simulink library "Lib_MCHP_BLKDEMO_Motor"  (R2015b)
settings: Solver=VariableStepAuto  StartTime=0.0  StopTime=10.0  RelTol=1e-3
values from neighbouring files (symbols this model uses):
  DEADTIME = 1e-6    (= 1e-06)    [UserParams.m]
  PSHIFT = TConv/2    (= 4.680375e-06)    [UserParams.m]
  PWMFREQUENCY = 20e3    (= 20000)    [UserParams.m]
  TSETTLE = 2e-6    (= 2e-06)    [UserParams.m]
  TSmp = 0.343*1e-6    (= 3.43e-07)    [UserParams.m]
undefined symbols (not defined in the file or in its folder): A4, B15, B9, C6, F0, P20, P41, P47, P54, P96, Pin, PWMmax, XData
libraries: MCHP_Blockset x9, simulink x7, Lib_MCHP_BLKDEMO_Motor x6
(part 1 of 2)
settings Model: Creator=M91449  LastModifiedBy=M91449

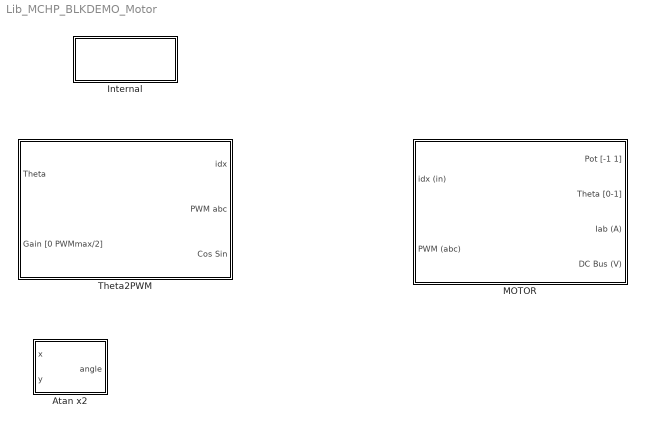
== system Lib_MCHP_BLKDEMO_Motor ==
  Atan x2 : Subsystem
  Internal : Subsystem
  MOTOR : Subsystem  Variant=on  OverrideUsingVariant=SingleShunt_CenterAligned
  Theta2PWM : Subsystem  Variant=on  VariantControl=Variant  OverrideUsingVariant=Optimized

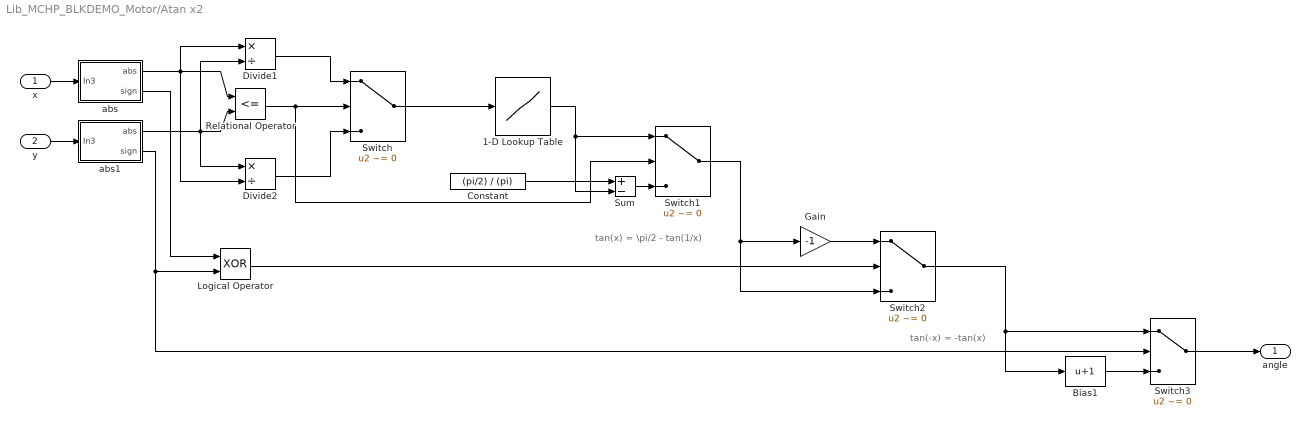
== system Lib_MCHP_BLKDEMO_Motor/Atan x2 ==
  note: tan(x) = \pi/2 - tan(1/x)
  note: tan(-x) = -tan(x)
  x : Inport
  y : Inport  Port=2
  1-D Lookup Table : Lookup_n-D  NumberOfTableDimensions=1  BreakpointsSpecification=Even spacing  BreakpointsForDimension1=[0:2^-8:1]  BreakpointsForDimension1FirstPoint=0  BreakpointsForDimension1Spacing=2^-8  IndexSearchMethod=Evenly spaced points  BeginIndexSearchUsingPreviousIndexResult=on  Table=atan([0:2^-8:1])/(pi)  TableDataTypeStr=fixdt(1,16,15)  InterpMethod=Flat  ExtrapMethod=Clip  RemoveProtectionInput=on  UseLastTableValue=on  OutDataTypeStr=fixdt(1,16,15)  RndMeth=Simplest  InputSameDT=on  LockScale=on
  Bias1 : Bias  Bias=1
  Constant : Constant  Value=(pi/2) / (pi)  OutDataTypeStr=Inherit: Inherit via back propagation
  Divide1 : Product  Inputs=*/  OutDataTypeStr=fixdt(0,16,15)
  Divide2 : Product  Inputs=*/  OutDataTypeStr=fixdt(0,16,15)
  Gain : Gain  Gain=-1  OutDataTypeStr=Inherit: Same as input
  Logical Operator : Logic  Operator=XOR  AllPortsSameDT=off  OutDataTypeStr=boolean
  Relational Operator : RelationalOperator  Operator=<=  OutDataTypeStr=boolean
  Sum : Sum  Inputs=+-
  Switch{,1..3} (4 alike) : Switch  Criteria=u2 ~= 0
  abs : Subsystem
  abs1 : Subsystem
  angle : Outport
  wires:
  Gain/1 -> Switch2/1
  Bias1/1 -> Switch3/3
  Switch3/1 -> angle/1
  Switch2/1 -> Switch3/1, Bias1/1
  Relational Operator/1 -> Switch/2, Switch1/2
  Divide2/1 -> Switch/3
  Divide1/1 -> Switch/1
  Switch/1 -> 1-D Lookup Table/1
  1-D Lookup Table/1 -> Switch1/1, Sum/2
  Constant/1 -> Sum/1
  Sum/1 -> Switch1/3
  abs/1(abs) -> Relational Operator/1, Divide1/1, Divide2/2
  x/1 -> abs/1(In3)
  abs1/1(abs) -> Relational Operator/2, Divide2/1, Divide1/2
  y/1 -> abs1/1(In3)
  abs/2(sign) -> Logical Operator/1
  abs1/2(sign) -> Logical Operator/2, Switch3/2
  Logical Operator/1 -> Switch2/2
  Switch1/1 -> Gain/1, Switch2/3

== system Lib_MCHP_BLKDEMO_Motor/Internal ==
  Trig : Subsystem

== system Lib_MCHP_BLKDEMO_Motor/MOTOR ==
  idx (in) : Inport
  PWM (abc) : Inport  Port=2
  DUAL SHUNT Center Aligned : Subsystem  VariantControl=(default)
  SINGLE SHUNT Center Aligned : Subsystem  VariantControl=SingleShunt_CenterAligned
  SINGLE SHUNT Edge Aligned : Subsystem  VariantControl=SingleShunt_EdgeAligned
  Pot [-1 1] : Outport
  Theta [0-1] : Outport  Port=2
  Iab (A) : Outport  Port=3
  DC Bus (V) : Outport  Port=4

== system Lib_MCHP_BLKDEMO_Motor/Theta2PWM ==
  Theta : Inport
  Gain [0 PWMmax/2] : Inport  Port=2
  Theta2PWM : Subsystem  VariantControl=(default)
  Theta2PWM Optimized : Subsystem  VariantControl=Optimized
  idx : Outport
  PWM abc : Outport  Port=2
  Cos Sin : Outport  Port=3

== system Lib_MCHP_BLKDEMO_Motor/Atan x2/abs ==
  In3 : Inport
  Compare To Zero : simulink/Logic and Bit Operations/Compare To Zero  relop=>=  OutDataTypeStr=boolean
  Gain : Gain  Gain=-1  OutDataTypeStr=Inherit: Same as input
  Switch2 : Switch  Criteria=u2 ~= 0
  abs : Outport
  sign : Outport  Port=2
  wires:
  Compare To Zero/1 -> Switch2/2, sign/1
  In3/1 -> Compare To Zero/1, Switch2/1, Gain/1
  Gain/1 -> Switch2/3
  Switch2/1 -> abs/1

== system Lib_MCHP_BLKDEMO_Motor/Atan x2/abs1 ==
  In3 : Inport
  Compare To Zero : simulink/Logic and Bit Operations/Compare To Zero  relop=>=  OutDataTypeStr=boolean
  Gain : Gain  Gain=-1  OutDataTypeStr=Inherit: Same as input
  Switch2 : Switch  Criteria=u2 ~= 0
  abs : Outport
  sign : Outport  Port=2
  wires:
  Switch2/1 -> abs/1
  Gain/1 -> Switch2/3
  In3/1 -> Gain/1, Switch2/1, Compare To Zero/1
  Compare To Zero/1 -> sign/1, Switch2/2

== system Lib_MCHP_BLKDEMO_Motor/Internal/Trig ==
  note: Compute ADC Trig point for Single Shunt Center Aligned Motor Control drive
  In1 : Inport
  Bias : Bias  Bias=65535-2*PWMmax
  Bias1 : Bias  Bias=65535-2*PWMmax
  Constant1 : Constant  Value=floor(PWMmax + (DEADTIME + TSETTLE - TSmp) * PWMmax * PWMFREQUENCY*2)  OutDataTypeStr=uint16
  Demux8 : Demux  Outputs=2
  Gain : Gain  OutDataTypeStr=Inherit: Same as input
  Mux43 : Mux  Inputs=2
  Sum7 : Sum  OutDataTypeStr=Inherit: Same as accumulator
  Switch : Switch  Criteria=u2 > Threshold  Threshold=2*PWMmax
  Switch1 : Switch  Criteria=u2 > Threshold  Threshold=2*PWMmax
  Out1 : Outport
  wires:
  Bias1/1 -> Switch1/1
  Bias/1 -> Switch/1
  Demux8/1 -> Mux43/1, Bias/1, Switch/2, Switch/3
  Demux8/2 -> Mux43/2, Bias1/1, Switch1/2, Switch1/3
  Gain/1 -> Demux8/1
  In1/1 -> Sum7/2
  Sum7/1 -> Gain/1
  Constant1/1 -> Sum7/1
  Mux43/1 -> Out1/1

== system Lib_MCHP_BLKDEMO_Motor/MOTOR/DUAL SHUNT Center Aligned ==
  idx (in) : Inport
  PWM (abc) : Inport  Port=2
  MOTOR Cmd : Subsystem
  MOTOR - Board Sensor : Subsystem
  Pot [-1 1] : Outport
  Theta [0-1] : Outport  Port=2
  Iab (A) : Outport  Port=3
  DC Bus (V) : Outport  Port=4
  wires:
  MOTOR - Board Sensor/3(Theta) -> Theta [0-1]/1
  MOTOR Cmd/1(idx out) -> MOTOR - Board Sensor/1(idx (in))
  MOTOR - Board Sensor/1(DC Bus (V)) -> DC Bus (V)/1
  MOTOR - Board Sensor/4(Pot) -> Pot [-1 1]/1
  PWM (abc)/1 -> MOTOR Cmd/2(PWM (abc))
  MOTOR - Board Sensor/2(Iab (A)) -> Iab (A)/1
  idx (in)/1 -> MOTOR Cmd/1(idx in)

== system Lib_MCHP_BLKDEMO_Motor/MOTOR/SINGLE SHUNT Center Aligned ==
  idx (in) : Inport
  PWM (abc) : Inport  Port=2
  MOTOR Cmd : Subsystem
  MOTOR - Board Sensor : Subsystem
  Pot [-1 1] : Outport
  Theta [0-1] : Outport  Port=2
  Iab (A) : Outport  Port=3
  DC Bus (V) : Outport  Port=4
  wires:
  idx (in)/1 -> MOTOR Cmd/1(idx in)
  MOTOR - Board Sensor/2(Iab (A)) -> Iab (A)/1
  PWM (abc)/1 -> MOTOR Cmd/2(PWM (abc))
  MOTOR - Board Sensor/4(Pot) -> Pot [-1 1]/1
  MOTOR - Board Sensor/1(DC Bus (V)) -> DC Bus (V)/1
  MOTOR Cmd/1(idx out) -> MOTOR - Board Sensor/1(idx (in))
  MOTOR - Board Sensor/3(Theta) -> Theta [0-1]/1

== system Lib_MCHP_BLKDEMO_Motor/MOTOR/SINGLE SHUNT Edge Aligned ==
  idx (in) : Inport
  PWM (abc) : Inport  Port=2
  MOTOR Cmd : Subsystem
  MOTOR - Board Sensor : Subsystem
  Pot [-1 1] : Outport
  Theta [0-1] : Outport  Port=2
  Iab (A) : Outport  Port=3
  DC Bus (V) : Outport  Port=4
  wires:
  idx (in)/1 -> MOTOR Cmd/1(idx in)
  MOTOR - Board Sensor/2(Iab (A)) -> Iab (A)/1
  PWM (abc)/1 -> MOTOR Cmd/2(PWM (abc))
  MOTOR - Board Sensor/4(Pot) -> Pot [-1 1]/1
  MOTOR - Board Sensor/1(DC Bus (V)) -> DC Bus (V)/1
  MOTOR Cmd/1(idx out) -> MOTOR - Board Sensor/1(idx (in))
  MOTOR - Board Sensor/3(Theta) -> Theta [0-1]/1

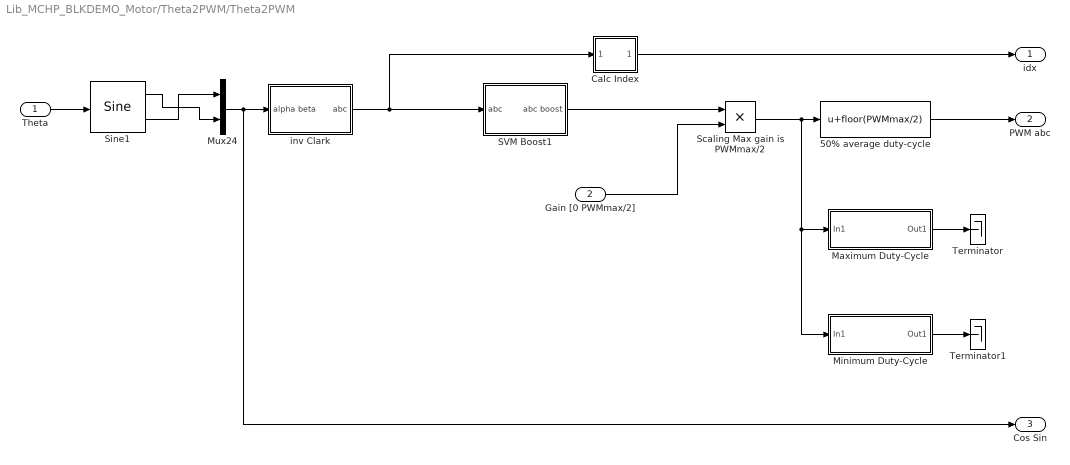
== system Lib_MCHP_BLKDEMO_Motor/Theta2PWM/Theta2PWM ==
  Theta : Inport  OutDataTypeStr=fixdt(0,16,16)
  Gain [0 PWMmax/2] : Inport  Port=2  OutMax=[PWMmax/2]
  50% average duty-cycle : Bias  Bias=floor(PWMmax/2)
  Calc Index : Subsystem
  Maximum Duty-Cycle : Subsystem
  Minimum Duty-Cycle : Subsystem
  Mux24 : Mux  Inputs=2
  SVM Boost1 : Subsystem
  Scaling Max gain is PWMmax/2 : Product  Inputs=**  OutDataTypeStr=uint16
  Sine1 : simulink/Lookup Tables/Sine  Formula=sin(2*pi*u) and cos(2*pi*u)  NumDataPoints=(2^5)+1  OutputWordLength=16  InternalRulePriority=Speed
  Terminator : Terminator
  Terminator1 : Terminator
  inv Clark : Subsystem
  idx : Outport
  PWM abc : Outport  Port=2
  Cos Sin : Outport  Port=3
  wires:
  Sine1/1 -> Mux24/2
  Theta/1 -> Sine1/1
  inv Clark/1(abc) -> Calc Index/1(In1), SVM Boost1/1(abc)
  Calc Index/1(Idx) -> idx/1
  SVM Boost1/1(abc boost) -> Scaling Max gain is PWMmax/2/1
  50% average duty-cycle/1 -> PWM abc/1
  Sine1/2 -> Mux24/1
  Gain [0 PWMmax/2]/1 -> Scaling Max gain is PWMmax/2/2
  Scaling Max gain is PWMmax/2/1 -> 50% average duty-cycle/1, Maximum Duty-Cycle/1(In1), Minimum Duty-Cycle/1(In1)
  Mux24/1 -> Cos Sin/1, inv Clark/1(alpha beta)
  Maximum Duty-Cycle/1(Out1) -> Terminator/1
  Minimum Duty-Cycle/1(Out1) -> Terminator1/1

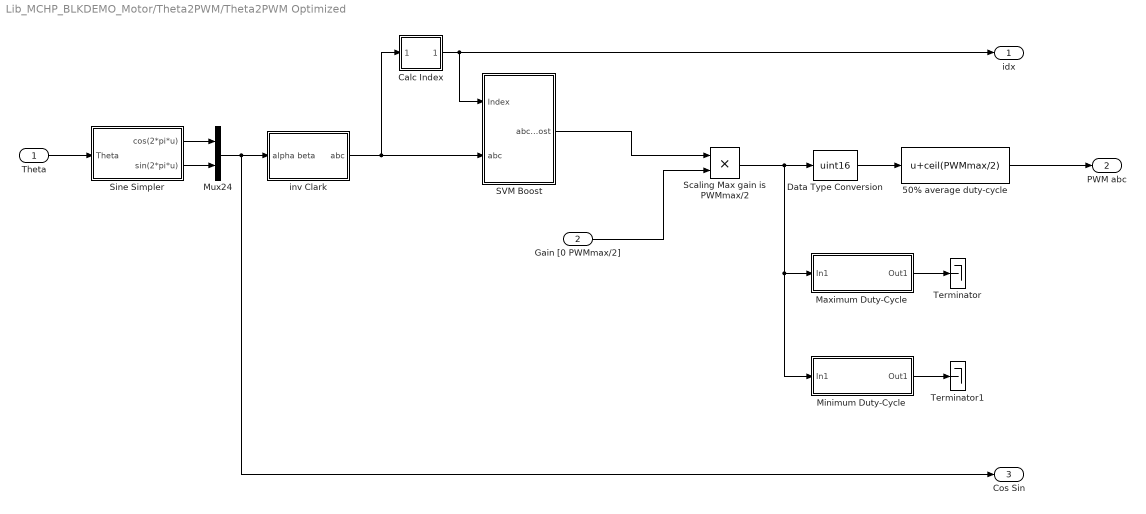
== system Lib_MCHP_BLKDEMO_Motor/Theta2PWM/Theta2PWM Optimized ==
  Theta : Inport  OutDataTypeStr=fixdt(0,16,16)
  Gain [0 PWMmax/2] : Inport  Port=2  OutMin=[-PWMmax/2]  OutMax=[PWMmax/2]
  50% average duty-cycle : Bias  Bias=ceil(PWMmax/2)
  Calc Index : Subsystem
  Data Type Conversion : DataTypeConversion  OutDataTypeStr=uint16  ConvertRealWorld=Stored Integer (SI)
  Maximum Duty-Cycle : Subsystem
  Minimum Duty-Cycle : Subsystem
  Mux24 : Mux  Inputs=2
  SVM Boost : Subsystem
  Scaling Max gain is PWMmax/2 : Product  Inputs=**  OutDataTypeStr=int16
  Sine Simpler : Subsystem
  Terminator : Terminator
  Terminator1 : Terminator
  inv Clark : Subsystem
  idx : Outport
  PWM abc : Outport  Port=2
  Cos Sin : Outport  Port=3
  wires:
  Data Type Conversion/1 -> 50% average duty-cycle/1
  50% average duty-cycle/1 -> PWM abc/1
  SVM Boost/1(abc boost) -> Scaling Max gain is PWMmax/2/1
  Sine Simpler/2(sin(2*pi*u)) -> Mux24/2
  Sine Simpler/1(cos(2*pi*u)) -> Mux24/1
  Theta/1 -> Sine Simpler/1(Theta)
  inv Clark/1(abc) -> SVM Boost/2(abc), Calc Index/1(In1)
  Calc Index/1(Idx) -> idx/1, SVM Boost/1(Index)
  Gain [0 PWMmax/2]/1 -> Scaling Max gain is PWMmax/2/2
  Scaling Max gain is PWMmax/2/1 -> Data Type Conversion/1, Maximum Duty-Cycle/1(In1), Minimum Duty-Cycle/1(In1)
  Maximum Duty-Cycle/1(Out1) -> Terminator/1
  Minimum Duty-Cycle/1(Out1) -> Terminator1/1
  Mux24/1 -> Cos Sin/1, inv Clark/1(alpha beta)

== system Lib_MCHP_BLKDEMO_Motor/MOTOR/DUAL SHUNT Center Aligned/MOTOR Cmd ==
  idx in : Inport
  PWM (abc) : Inport  Port=2
  Dead time Compensation : Bias  Bias=round( (2e-6/5e-5) *PWMmax )
  Demux : Demux  Outputs=3
  PWM High Speed : MCHP_Blockset/PWM IO/PWM High Speed  pop1=[1]  chk1="[1  1  1  0]"  chkHL1="[1  1  1  1  1  1  1 ; 1  1  1  1  1  1  1]"  maxP1="[5e-05       5e-05       5e-05       0.001       0.001       0.001       0.001 ; 0.001       0.001       1e-06       0.001       0.001       0.001       0.001]"  InitP2="[5e-05       5e-05       5e-05       0.001       0.001       0.001       0.001 ; 0.001       0.001       0.001       0.001       0.001       0.001       0.001]"  chkP2="[0  0  0  1  1  1  1 ; 1  0  0  1  1  1  1]"  InitDC="[4   4   4  50  50  50  50 ; 0.001        0.001        0.001           50           50           50           50]"  chkDC="[1  1  1  1  1  1  1 ; 0  0  0  1  1  1  1]"  InitPh="[0           0           0       0.001       0.001       0.001       0.001 ; 0           0           0       0.001       0.001       0.001       0.001]"  chkPh="[0  0  0  1  1  1  1 ; 0  0  0  1  1  1  1]"  edSEvTrigx={'0','-1','-1','-1','-1','-1','-1'}  chkSEvTrigx="[0  0  0  1  1  1  1]"  popFlt="[2  2  2  1  1  1  1]"  popFltPin="[20  20  20   4   4   4   4]"  popFltPinRp="[1  1  1  1  1  1  1]"  popFltActivH="[2  2  2  1  1  1  1]"  popFltForceH="[2  2  2  2  2  2  2]"  popFltForceL="[1  1  1  1  1  1  1]"  chkFltBlkOut="[0  0  0  0  0  0  0]"  popDT="[1  1  1  3  3  3  3]"  edDTRx="[0           0           0       1e-05       1e-05       1e-05       1e-05]"  edAltDTRx="[2e-06       2e-06       2e-06       1e-05       1e-05       1e-05       1e-05]"  S_INPUT="[5  5  5]"  S_INPUT_Size="[1  1  1]"  S_OUTPUT=[]  S_OUTPUT_Size=[]  S_DWORK_Type=[]  S_DWORK_Size=[]  ADC_VARTRIG={PWM Primary Special Event Trigger;6}  SampleTime=-1  ORDERING=None  MCHP_PORT={PWM1 Fault}{FLT32}4:0:B4;{PWM2 Fault}{FLT32}4:0:B4;{PWM3 Fault}{FLT32}4:0:B4;{PWM1H}{PWM1H}4:4:B14;{PWM1L}{PWM1L}4:4:B15;{PWM2H}{PWM2H}4:4:B12;{PWM2L}{PWM2L}4:4:B13;{PWM3H}{PWM3H}4:4:B10;{PWM3L}{PWM3L}4:4:B11;  MCHP_MASTERLINK=AN1078_33EP256MC506_ClosedLoop/Microchip Master  MCHP_VERSION=v3.38
  Saturation low side turn on errate workaround + errata for Phase shift (times 2) : Saturate  UpperLimit=PWMmax  LowerLimit=round( (2e-6/5e-5) *PWMmax )* 2
  int to uint : DataTypeConversion  OutDataTypeStr=uint16  ConvertRealWorld=Stored Integer (SI)
  idx out : Outport
  wires:
  PWM (abc)/1 -> Dead time Compensation/1
  Dead time Compensation/1 -> int to uint/1
  Saturation low side turn on errate workaround + errata for Phase shift (times 2)/1 -> Demux/1
  int to uint/1 -> Saturation low side turn on errate workaround + errata for Phase shift (times 2)/1
  Demux/2 -> PWM High Speed/2
  Demux/3 -> PWM High Speed/3
  Demux/1 -> PWM High Speed/1
  idx in/1 -> idx out/1

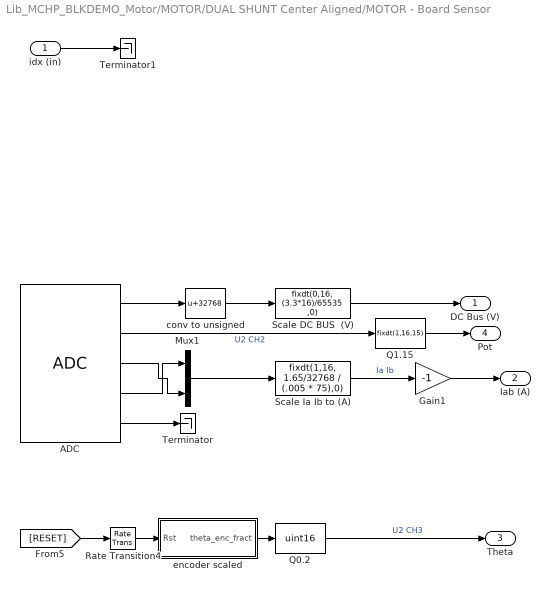
== system Lib_MCHP_BLKDEMO_Motor/MOTOR/DUAL SHUNT Center Aligned/MOTOR - Board Sensor ==
  idx (in) : Inport
  ADC : MCHP_Blockset/Analog IO/ADC  Priority=5  ADC_REF=1  Mode=10 bits (allows exact simultaneous sampling)  FORM="sddd dddd dddd 0000  ==> Signed fractional"  nSAMPLECHANNELS=CH0 : CH1 : CH2 : CH3  nSAMPLECHANNELS_12bits=CH0 only  SIMULTANEOUS=Simultaneously on all Channels  ADxCSS=[10 13]  MUXA_CH0N=off  MUXA_CH123=Dynamic Options  MUXA_CH123_TXT=AN0 : AN1 : AN2  MUXB_CH0=AN1  MUXB_CH0N=on  MUXB_CH123=Dynamic Options  MUXB_CH123_TXT=AN0 : AN1 : AN2  SequenceRepeat=1  SequenceTiming=are done as fast as possible ; triggered by user define source  SSRC_SSRCG=Dynamic Options  SSRC_SSRCG_TXT=6  Update_BlockOutput=After each trig and conversion sequence  Trig_TimeStep=with each update of the ADC block output  ADC_DMA_CHANNEL=Use Interrupt instead of DMA  SampleTime=5e-05  Info=Total Time for Sample & Conversion : 8.9143e-06s including 3.4286e-07s (x 2) sample time.  MCHP_PORT={Analog Input 0}{AN0}15:2:A0;{Analog Input 1}{AN1}15:2:A1;{Analog Input 2}{AN2}15:2:B0;{Analog Input 10}{AN10}15:2:A12;{Analog Input 13}{AN13}15:2:E13;  MCHP_MASTERLINK=Test_PWMHS_33EP256MC506/Microchip Master  ADC_TIMING=[8.9142857142857144e-06]
  Gain1 : Gain  Gain=-1  SaturateOnIntegerOverflow=on  OutDataTypeStr=Inherit: Same as input
  Mux1 : Mux  Inputs=2
  Q0.2 : DataTypeConversion  OutDataTypeStr=uint16  ConvertRealWorld=Stored Integer (SI)
  Q1.15 : DataTypeConversion  OutDataTypeStr=fixdt(1,16,15)  ConvertRealWorld=Stored Integer (SI)
  Rate Transition4 : RateTransition  X0=1
  Scale DC BUS  (V) : DataTypeConversion  OutDataTypeStr=fixdt(0,16, (3.3*16)/65535 ,0)  ConvertRealWorld=Stored Integer (SI)
  Scale Ia Ib to (A) : DataTypeConversion  OutDataTypeStr=fixdt(1,16, 1.65/32768 / (.005 * 75),0)  ConvertRealWorld=Stored Integer (SI)
  Terminator : Terminator
  Terminator1 : Terminator
  conv to unsigned : Bias  Bias=32768
  encoder scaled : Subsystem
  DC Bus (V) : Outport
  Iab (A) : Outport  Port=2
  Theta : Outport  Port=3
  Pot : Outport  Port=4
  wires:
  ADC/5 -> Terminator/1
  Rate Transition4/1 -> encoder scaled/1(Rst)
  ADC/1 -> conv to unsigned/1
  Mux1/1 -> Scale Ia Ib to (A)/1
  conv to unsigned/1 -> Scale DC BUS  (V)/1
  ADC/4 -> Mux1/1
  ADC/3 -> Mux1/2
  encoder scaled/1(theta_enc_fract) -> Q0.2/1
  [RESET] -> Rate Transition4/1
  ADC/2 -> Q1.15/1  "U2 CH2"
  Q0.2/1 -> Theta/1  "U2 CH3"
  Scale Ia Ib to (A)/1 -> Gain1/1  "Ia Ib"
  Scale DC BUS  (V)/1 -> DC Bus (V)/1
  Gain1/1 -> Iab (A)/1
  idx (in)/1 -> Terminator1/1
  Q1.15/1 -> Pot/1

== system Lib_MCHP_BLKDEMO_Motor/MOTOR/SINGLE SHUNT Center Aligned/MOTOR Cmd ==
  idx in : Inport
  PWM (abc) : Inport  Port=2
  Demux2 : Demux
  PWM High Speed : MCHP_Blockset/PWM IO/PWM High Speed  pop1=[1]  chk1="[1  1  1  0  1]"  chkHL1="[1  1  1  1  1  1  1 ; 1  1  1  1  1  1  1]"  maxP1={ '1/PWMFREQUENCY','5e-05','5e-05','0.001','0.001','0.001','0.001';'0.001','0.001','1e-06','0.001','0.001','0.001','0.001'}  InitP2={ '1/PWMFREQUENCY','5e-05','5e-05','0.001','0.001','0.001','0.001';'0.001','0.001','0.001','0.001','0.001','0.001','0.001'}  chkP2="[0  0  0  1  1  1  1 ; 1  0  0  1  1  1  1]"  InitDC={ '[50 50]','[50 50]','[50 50]','[5 5]','[5 5]','[5 5]','[5 5]';'[0 0]','[0 0]','[0 0]','[5 5]','[5 5]','[5 5]','[5 5]'}  chkDC="[1  1  1  1  1  1  1 ; 0  0  0  1  1  1  1]"  InitPh={ 'DEADTIME','DEADTIME','DEADTIME','0.001','0.001','0.001','0.001';'0','0','0','0.001','0.001','0.001','0.001'}  chkPh="[1  1  1  1  1  1  1 ; 0  0  0  1  1  1  1]"  edSEvTrigx="{ '[1/(2*PWMFREQUENCY)+PSHIFT  1/(2*PWMFREQUENCY) + PSHIFT*2]','-1','-1','-1','-1','-1','-1'}"  chkSEvTrigx="[1  0  0  1  1  1  1]"  popFlt="[2  2  2  1  1  1  1]"  popFltPin="[20  20  20   4   4   4   4]"  popFltPinRp="[1  1  1  1  1  1  1]"  popFltActivH="[2  2  2  1  1  1  1]"  popFltForceH="[2  2  2  2  2  2  2]"  popFltForceL="[1  1  1  1  1  1  1]"  chkFltBlkOut="[0  0  0  0  0  0  0]"  popDT="[1  1  1  3  3  3  3]"  edDTRx={ 'DEADTIME','DEADTIME','DEADTIME','1e-05','1e-05','1e-05','1e-05'}  edAltDTRx={ 'DEADTIME','DEADTIME','DEADTIME','1e-05','1e-05','1e-05','1e-05'}  S_INPUT="[5  5  5  5]"  S_INPUT_Size="[2  2  2  2]"  S_OUTPUT=[]  S_OUTPUT_Size=[]  S_DWORK_Type="[5  5  5  5]"  S_DWORK_Size="[1  12   1   2]"  ADC_VARTRIG={PWM Primary Special Event Trigger;6}  SampleTime=-1  ORDERING=None  MCHP_PORT={PWM1 Fault}{FLT32}4:0:B4;{PWM2 Fault}{FLT32}4:0:B4;{PWM3 Fault}{FLT32}4:0:B4;{PWM1H}{PWM1H}4:4:B14;{PWM1L}{PWM1L}4:4:B15;{PWM2H}{PWM2H}4:4:B12;{PWM2L}{PWM2L}4:4:B13;{PWM3H}{PWM3H}4:4:B10;{PWM3L}{PWM3L}4:4:B11;  MCHP_MASTERLINK=Test_PWMHS_33EP256MC506/Microchip Master  MCHP_VERSION=v3.38
  Phase Shift & Trig Point : Subsystem
  Saturation low side turn on errate workaround + errata for Phase shift (times 2)1 : Saturate  UpperLimit=PWMmax - PSHIFT * PWMmax * PWMFREQUENCY * 2  LowerLimit=PSHIFT * PWMmax * PWMFREQUENCY * 2
  int to uint : DataTypeConversion  OutDataTypeStr=uint16  ConvertRealWorld=Stored Integer (SI)
  idx out : Outport
  wires:
  idx in/1 -> Phase Shift & Trig Point/1(Index), idx out/1
  PWM (abc)/1 -> int to uint/1
  int to uint/1 -> Saturation low side turn on errate workaround + errata for Phase shift (times 2)1/1
  Saturation low side turn on errate workaround + errata for Phase shift (times 2)1/1 -> Phase Shift & Trig Point/2(In1)
  Demux2/1 -> PWM High Speed/1
  Demux2/2 -> PWM High Speed/2
  Demux2/3 -> PWM High Speed/3
  Demux2/4 -> PWM High Speed/4
  Phase Shift & Trig Point/1(Out1) -> Demux2/1

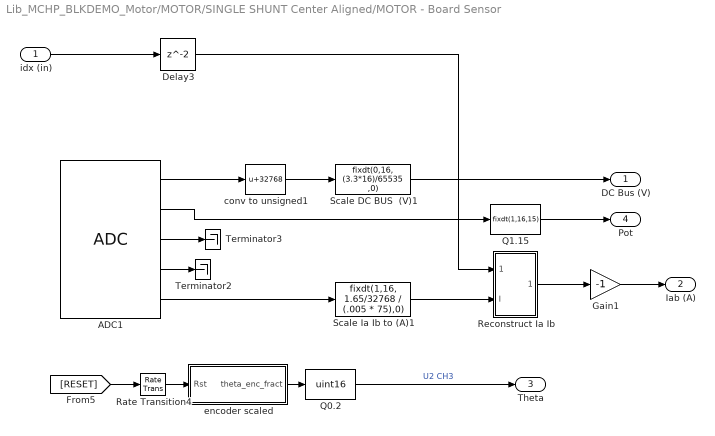
== system Lib_MCHP_BLKDEMO_Motor/MOTOR/SINGLE SHUNT Center Aligned/MOTOR - Board Sensor ==
  idx (in) : Inport
  ADC1 : MCHP_Blockset/Analog IO/ADC  Priority=5  ADC_REF=1  Mode=10 bits (allows exact simultaneous sampling)  FORM="sddd dddd dddd 0000  ==> Signed fractional"  nSAMPLECHANNELS=CH0 : CH1 : CH2 : CH3  nSAMPLECHANNELS_12bits=CH0 only  SIMULTANEOUS=Simultaneously on all Channels  ADxCSS=[10 13]  MUXA_CH0N=off  MUXA_CH123=Dynamic Options  MUXA_CH123_TXT=AN0 : AN1 : AN2  MUXB_CH0=AN1  MUXB_CH0N=on  MUXB_CH123=Dynamic Options  MUXB_CH123_TXT=AN0 : AN1 : AN2  SequenceRepeat=1  SequenceTiming=are done as fast as possible ; triggered by user define source  SSRC_SSRCG=Dynamic Options  SSRC_SSRCG_TXT=6  Update_BlockOutput=After all trig and conversion sequence  Trig_TimeStep=with each update of the ADC block output  ADC_DMA_CHANNEL=Use Interrupt instead of DMA  SampleTime=5e-05  Info=Total Time for Sample & Conversion : 8.9143e-06s including 3.4286e-07s (x 2) sample time.  MCHP_PORT={Analog Input 0}{AN0}15:2:A0;{Analog Input 1}{AN1}15:2:A1;{Analog Input 2}{AN2}15:2:B0;{Analog Input 10}{AN10}15:2:A12;{Analog Input 13}{AN13}15:2:E13;  MCHP_MASTERLINK=Test_PWMHS_33EP256MC506/Microchip Master  ADC_TIMING=[8.9142857142857144e-06]
  Delay3 : Delay  InitialCondition=0
  Gain1 : Gain  Gain=-1  OutDataTypeStr=Inherit: Same as input
  Q0.2 : DataTypeConversion  OutDataTypeStr=uint16  ConvertRealWorld=Stored Integer (SI)
  Q1.15 : DataTypeConversion  OutDataTypeStr=fixdt(1,16,15)  ConvertRealWorld=Stored Integer (SI)
  Rate Transition4 : RateTransition  X0=1
  Reconstruct Ia Ib : Subsystem
  Scale DC BUS  (V)1 : DataTypeConversion  OutDataTypeStr=fixdt(0,16, (3.3*16)/65535 ,0)  ConvertRealWorld=Stored Integer (SI)
  Scale Ia Ib to (A)1 : DataTypeConversion  OutDataTypeStr=fixdt(1,16, 1.65/32768 / (.005 * 75),0)  ConvertRealWorld=Stored Integer (SI)
  Terminator2 : Terminator
  Terminator3 : Terminator
  conv to unsigned1 : Bias  Bias=32768
  encoder scaled : Subsystem
  DC Bus (V) : Outport
  Iab (A) : Outport  Port=2
  Theta : Outport  Port=3
  Pot : Outport  Port=4
  wires:
  Rate Transition4/1 -> encoder scaled/1(Rst)
  encoder scaled/1(theta_enc_fract) -> Q0.2/1
  [RESET] -> Rate Transition4/1
  Q0.2/1 -> Theta/1  "U2 CH3"
  ADC1/5 -> Scale Ia Ib to (A)1/1
  Scale Ia Ib to (A)1/1 -> Reconstruct Ia Ib/2(I)
  idx (in)/1 -> Delay3/1
  Delay3/1 -> Reconstruct Ia Ib/1(Index)
  ADC1/3 -> Terminator3/1
  ADC1/1 -> conv to unsigned1/1
  conv to unsigned1/1 -> Scale DC BUS  (V)1/1
  Scale DC BUS  (V)1/1 -> DC Bus (V)/1
  Reconstruct Ia Ib/1(Ia Ib) -> Gain1/1
  Gain1/1 -> Iab (A)/1
  ADC1/2 -> Q1.15/1
  ADC1/4 -> Terminator2/1
  Q1.15/1 -> Pot/1

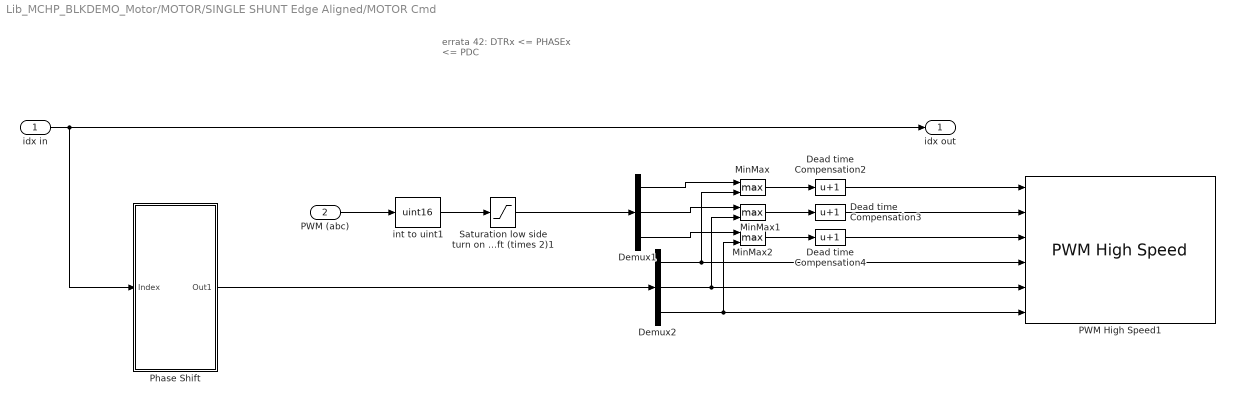
== system Lib_MCHP_BLKDEMO_Motor/MOTOR/SINGLE SHUNT Edge Aligned/MOTOR Cmd ==
  note: errata 42:
      | DTRx <= PHASEx <= PDC
  idx in : Inport
  PWM (abc) : Inport  Port=2
  Dead time Compensation2 : Bias  Bias=1
  Dead time Compensation3 : Bias  Bias=1
  Dead time Compensation4 : Bias  Bias=1
  Demux1 : Demux  Outputs=3
  Demux2 : Demux  Outputs=3
  MinMax : MinMax  Function=max  Inputs=2
  MinMax1 : MinMax  Function=max  Inputs=2
  MinMax2 : MinMax  Function=max  Inputs=2
  PWM High Speed1 : MCHP_Blockset/PWM IO/PWM High Speed  pop1=[1]  chk1="[0  1  0  0  0]"  chkHL1="[1  1  1  1  1  1  1 ; 1  1  1  1  1  1  1]"  maxP1={ '1/PWMFREQUENCY','5e-05','5e-05','0.001','0.001','0.001','0.001';'0.001','0.001','1e-06','0.001','0.001','0.001','0.001'}  InitP2={ '1/PWMFREQUENCY','5e-05','5e-05','0.001','0.001','0.001','0.001';'0.001','0.001','0.001','0.001','0.001','0.001','0.001'}  chkP2="[0  0  0  1  1  1  1 ; 1  0  0  1  1  1  1]"  InitDC={ '50','50','50','50','50','50','50';'0.001','0.001','0.001','50','50','50','50'}  chkDC="[1  1  1  1  1  1  1 ; 0  0  0  1  1  1  1]"  InitPh={ 'DEADTIME','DEADTIME','DEADTIME','0.001','0.001','0.001','0.001';'0','0','0','0.001','0.001','0.001','0.001'}  chkPh="[1  1  1  1  1  1  1 ; 0  0  0  1  1  1  1]"  edSEvTrigx={ 'TRIGS','-1','-1','-1','-1','-1','-1'}  chkSEvTrigx="[0  0  0  1  1  1  1]"  popFlt="[2  2  2  1  1  1  1]"  popFltPin="[20  20  20   4   4   4   4]"  popFltPinRp="[1  1  1  1  1  1  1]"  popFltActivH="[2  2  2  1  1  1  1]"  popFltForceH="[2  2  2  2  2  2  2]"  popFltForceL="[1  1  1  1  1  1  1]"  chkFltBlkOut="[0  0  0  0  0  0  0]"  popDT="[1  1  1  3  3  3  3]"  edDTRx={ 'DEADTIME','DEADTIME','DEADTIME','1e-05','1e-05','1e-05','1e-05'}  edAltDTRx={ 'DEADTIME','DEADTIME','DEADTIME','1e-05','1e-05','1e-05','1e-05'}  S_INPUT="[5  5  5  5  5  5]"  S_INPUT_Size="[1  1  1  1  1  1]"  S_OUTPUT=[]  S_OUTPUT_Size=[]  S_DWORK_Type=[5]  S_DWORK_Size=[1]  ADC_VARTRIG={PWM Primary Special Event Trigger;6}  SampleTime=-1  ORDERING=None  MCHP_PORT={PWM1 Fault}{FLT32}4:0:B4;{PWM2 Fault}{FLT32}4:0:B4;{PWM3 Fault}{FLT32}4:0:B4;{PWM1H}{PWM1H}4:4:B14;{PWM1L}{PWM1L}4:4:B15;{PWM2H}{PWM2H}4:4:B12;{PWM2L}{PWM2L}4:4:B13;{PWM3H}{PWM3H}4:4:B10;{PWM3L}{PWM3L}4:4:B11;  MCHP_MASTERLINK=Test_PWMHS_33EP256MC506/Microchip Master  MCHP_VERSION=v3.38
  Phase Shift : Subsystem
  Saturation low side turn on errate workaround + errata for Phase shift (times 2)1 : Saturate  UpperLimit=PWMmax-2  LowerLimit=ceil((DEADTIME * PWMFREQUENCY * PWMmax)/2)
  int to uint1 : DataTypeConversion  OutDataTypeStr=uint16  ConvertRealWorld=Stored Integer (SI)
  idx out : Outport
  wires:
  Dead time Compensation4/1 -> PWM High Speed1/3
  Dead time Compensation3/1 -> PWM High Speed1/2
  Dead time Compensation2/1 -> PWM High Speed1/1
  PWM (abc)/1 -> int to uint1/1
  int to uint1/1 -> Saturation low side turn on errate workaround + errata for Phase shift (times 2)1/1
  idx in/1 -> Phase Shift/1(Index), idx out/1
  Phase Shift/1(Out1) -> Demux2/1
  Demux2/2 -> PWM High Speed1/5, MinMax1/2
  Demux2/3 -> PWM High Speed1/6, MinMax2/2
  Saturation low side turn on errate workaround + errata for Phase shift (times 2)1/1 -> Demux1/1
  Demux2/1 -> PWM High Speed1/4, MinMax/2
  Demux1/1 -> MinMax/1
  MinMax/1 -> Dead time Compensation2/1
  MinMax1/1 -> Dead time Compensation3/1
  Demux1/2 -> MinMax1/1
  MinMax2/1 -> Dead time Compensation4/1
  Demux1/3 -> MinMax2/1

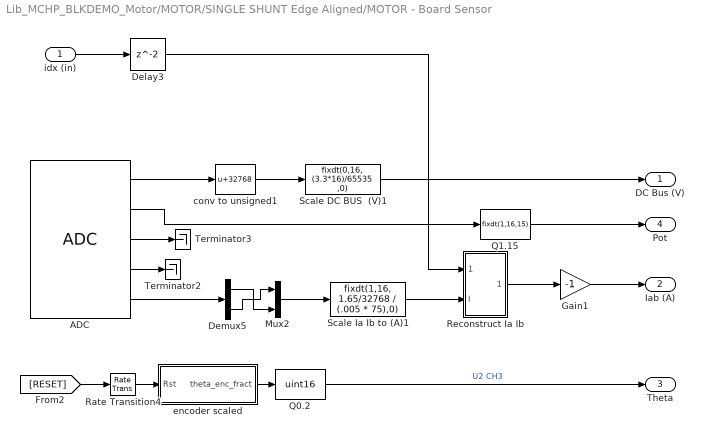
== system Lib_MCHP_BLKDEMO_Motor/MOTOR/SINGLE SHUNT Edge Aligned/MOTOR - Board Sensor ==
  idx (in) : Inport
  ADC : MCHP_Blockset/Analog IO/ADC  Priority=5  ADC_REF=1  Mode=10 bits (allows exact simultaneous sampling)  FORM="sddd dddd dddd 0000  ==> Signed fractional"  nSAMPLECHANNELS=CH0 : CH1 : CH2 : CH3  nSAMPLECHANNELS_12bits=CH0 only  SIMULTANEOUS=Simultaneously on all Channels  ADxCSS=[10 13]  MUXA_CH0N=off  MUXA_CH123=Dynamic Options  MUXA_CH123_TXT=AN0 : AN1 : AN2  MUXB_CH0=AN1  MUXB_CH0N=on  MUXB_CH123=Dynamic Options  MUXB_CH123_TXT=AN0 : AN1 : AN2  SequenceRepeat=1  SequenceTiming=are done as fast as possible ; triggered by user define source  SSRC_SSRCG=Dynamic Options  SSRC_SSRCG_TXT=6  Update_BlockOutput=After all trig and conversion sequence  Trig_TimeStep=with each update of the ADC block output  ADC_DMA_CHANNEL=Use Interrupt instead of DMA  SampleTime=5e-05  Info=Total Time for Sample & Conversion : 8.9143e-06s including 3.4286e-07s (x 2) sample time.  MCHP_PORT={Analog Input 0}{AN0}15:2:A0;{Analog Input 1}{AN1}15:2:A1;{Analog Input 2}{AN2}15:2:B0;{Analog Input 10}{AN10}15:2:A12;{Analog Input 13}{AN13}15:2:E13;  MCHP_MASTERLINK=Test_PWMHS_33EP256MC506/Microchip Master  ADC_TIMING=[8.9142857142857144e-06]
  Delay3 : Delay  InitialCondition=0
  Demux5 : Demux  Outputs=2
  Gain1 : Gain  Gain=-1  OutDataTypeStr=Inherit: Same as input
  Mux2 : Mux  Inputs=2
  Q0.2 : DataTypeConversion  OutDataTypeStr=uint16  ConvertRealWorld=Stored Integer (SI)
  Q1.15 : DataTypeConversion  OutDataTypeStr=fixdt(1,16,15)  ConvertRealWorld=Stored Integer (SI)
  Rate Transition4 : RateTransition  X0=1
  Reconstruct Ia Ib : Subsystem
  Scale DC BUS  (V)1 : DataTypeConversion  OutDataTypeStr=fixdt(0,16, (3.3*16)/65535 ,0)  ConvertRealWorld=Stored Integer (SI)
  Scale Ia Ib to (A)1 : DataTypeConversion  OutDataTypeStr=fixdt(1,16, 1.65/32768 / (.005 * 75),0)  ConvertRealWorld=Stored Integer (SI)
  Terminator2 : Terminator
  Terminator3 : Terminator
  conv to unsigned1 : Bias  Bias=32768
  encoder scaled : Subsystem
  DC Bus (V) : Outport
  Iab (A) : Outport  Port=2
  Theta : Outport  Port=3
  Pot : Outport  Port=4
  wires:
  Rate Transition4/1 -> encoder scaled/1(Rst)
  encoder scaled/1(theta_enc_fract) -> Q0.2/1
  [RESET] -> Rate Transition4/1
  Q0.2/1 -> Theta/1  "U2 CH3"
  Scale Ia Ib to (A)1/1 -> Reconstruct Ia Ib/2(I)
  idx (in)/1 -> Delay3/1
  Reconstruct Ia Ib/1(Ia Ib) -> Gain1/1
  Delay3/1 -> Reconstruct Ia Ib/1(Index)
  ADC/3 -> Terminator3/1
  ADC/1 -> conv to unsigned1/1
  conv to unsigned1/1 -> Scale DC BUS  (V)1/1
  Scale DC BUS  (V)1/1 -> DC Bus (V)/1
  Demux5/1 -> Mux2/2
  Demux5/2 -> Mux2/1
  Mux2/1 -> Scale Ia Ib to (A)1/1
  ADC/5 -> Demux5/1
  Gain1/1 -> Iab (A)/1
  ADC/2 -> Q1.15/1
  ADC/4 -> Terminator2/1
  Q1.15/1 -> Pot/1

== system Lib_MCHP_BLKDEMO_Motor/Theta2PWM/Theta2PWM/Calc Index ==
  In1 : Inport
  Bitwise Operator1 : simulink/Logic and Bit Operations/Bitwise Operator  logicop=OR  UseBitMask=off  NumInputPorts=3  BitMask=bin2dec('11011001')  BitMaskRealWorld=Stored Integer
  Data Type Conversion : DataTypeConversion  OutDataTypeStr=uint16  ConvertRealWorld=Stored Integer (SI)
  Demux1 : Demux  Outputs=3
  Gain6 : Gain  Gain=4  OutDataTypeStr=Inherit: Same as input
  Gain7 : Gain  Gain=2  OutDataTypeStr=Inherit: Same as input
  Relational Operator3 : RelationalOperator  Operator=>  OutDataTypeStr=fixdt(1,16)
  Relational Operator4 : RelationalOperator  Operator=>  OutDataTypeStr=fixdt(1,16)
  Relational Operator5 : RelationalOperator  Operator=>  OutDataTypeStr=fixdt(1,16)
  Idx : Outport
  wires:
  Data Type Conversion/1 -> Idx/1
  In1/1 -> Demux1/1
  Bitwise Operator1/1 -> Data Type Conversion/1
  Demux1/1 -> Relational Operator3/1, Relational Operator4/1
  Relational Operator4/1 -> Gain7/1
  Demux1/3 -> Relational Operator4/2, Relational Operator5/2
  Demux1/2 -> Relational Operator3/2, Relational Operator5/1
  Relational Operator3/1 -> Gain6/1
  Relational Operator5/1 -> Bitwise Operator1/3
  Gain6/1 -> Bitwise Operator1/1
  Gain7/1 -> Bitwise Operator1/2

== system Lib_MCHP_BLKDEMO_Motor/Theta2PWM/Theta2PWM/Maximum Duty-Cycle ==
  In1 : Inport
  Constant1 : Constant  Value=PWMmax  OutDataTypeStr=uint16
  MinMax1 : MinMax  Function=max  OutDataTypeStr=int16  InputSameDT=on
  Sum1 : Sum  Inputs=+-  AccumDataTypeStr=uint16  OutDataTypeStr=Inherit: Same as accumulator  RndMeth=Simplest
  Sum2 : Sum  Inputs=|++  AccumDataTypeStr=uint16  OutDataTypeStr=Inherit: Same as accumulator  RndMeth=Simplest
  Out1 : Outport
  wires:
  Constant1/1 -> Sum1/1
  MinMax1/1 -> Sum1/2
  In1/1 -> Sum2/1, MinMax1/1
  Sum2/1 -> Out1/1
  Sum1/1 -> Sum2/2

== system Lib_MCHP_BLKDEMO_Motor/Theta2PWM/Theta2PWM/Minimum Duty-Cycle ==
  In1 : Inport
  Bias : Bias  Bias=-round( (2e-6/5e-5) *PWMmax )
  MinMax1 : MinMax  OutDataTypeStr=int16  InputSameDT=on
  Sum2 : Sum  Inputs=|+-  AccumDataTypeStr=uint16  OutDataTypeStr=Inherit: Same as accumulator  RndMeth=Simplest
  Out1 : Outport
  wires:
  In1/1 -> MinMax1/1, Sum2/1
  Sum2/1 -> Out1/1
  MinMax1/1 -> Bias/1
  Bias/1 -> Sum2/2

== system Lib_MCHP_BLKDEMO_Motor/Theta2PWM/Theta2PWM/SVM Boost1 ==
  abc : Inport
  Add : Sum  OutDataTypeStr=Inherit: Same as accumulator
  Add1 : Sum  Inputs=-+  OutDataTypeStr=Inherit: Same as accumulator
  Gain5 : Gain  Gain=0.5  RndMeth=Simplest  OutDataTypeStr=Inherit: Same as input
  Gain8 : Gain  Gain=2/sqrt(3)  OutDataTypeStr=Inherit: Same as input
  MinMax1 : MinMax  SaturateOnIntegerOverflow=on  InputSameDT=on
  MinMax2 : MinMax  Function=max  SaturateOnIntegerOverflow=on  InputSameDT=on
  abc boost : Outport
  wires:
  MinMax1/1 -> Add/1
  MinMax2/1 -> Add/2
  Add/1 -> Gain5/1
  Gain5/1 -> Add1/1
  Add1/1 -> Gain8/1
  abc/1 -> MinMax1/1, Add1/2, MinMax2/1
  Gain8/1 -> abc boost/1

== system Lib_MCHP_BLKDEMO_Motor/Theta2PWM/Theta2PWM/inv Clark ==
  note: k = 2/3 : invariant Magnitude
  note: Transposed version is better optimized with DSP (optional)
      | No impact on no DSP version
  alpha beta : Inport
  Clarke1 : Product  Multiplication=Matrix(*)  RndMeth=Simplest  OutDataTypeStr=Inherit: Same as first input
  Constant Magnitude : Constant  Value=[1 0 ; -1/2 sqrt(3)/2 ;-1/2 -sqrt(3)/2]'  OutDataTypeStr=Inherit: Inherit via back propagation  SampleTime=-1
  Math Function : Math  Operator=transpose  SaturateOnIntegerOverflow=on
  abc : Outport
  wires:
  Clarke1/1 -> abc/1
  Math Function/1 -> Clarke1/1
  alpha beta/1 -> Math Function/1
  Constant Magnitude/1 -> Clarke1/2

== system Lib_MCHP_BLKDEMO_Motor/Theta2PWM/Theta2PWM Optimized/Calc Index ==
  In1 : Inport
  Bitwise Operator1 : simulink/Logic and Bit Operations/Bitwise Operator  logicop=OR  UseBitMask=off  NumInputPorts=3  BitMask=bin2dec('11011001')  BitMaskRealWorld=Stored Integer
  Data Type Conversion : DataTypeConversion  OutDataTypeStr=uint16  ConvertRealWorld=Stored Integer (SI)
  Demux1 : Demux  Outputs=3
  Gain6 : Gain  Gain=4  OutDataTypeStr=Inherit: Same as input
  Gain7 : Gain  Gain=2  OutDataTypeStr=Inherit: Same as input
  Relational Operator3 : RelationalOperator  Operator=>  OutDataTypeStr=fixdt(1,16)
  Relational Operator4 : RelationalOperator  Operator=>  OutDataTypeStr=fixdt(1,16)
  Relational Operator5 : RelationalOperator  Operator=>  OutDataTypeStr=fixdt(1,16)
  Idx : Outport
  wires:
  Data Type Conversion/1 -> Idx/1
  In1/1 -> Demux1/1
  Bitwise Operator1/1 -> Data Type Conversion/1
  Demux1/1 -> Relational Operator3/1, Relational Operator4/1
  Relational Operator4/1 -> Gain7/1
  Demux1/3 -> Relational Operator4/2, Relational Operator5/2
  Demux1/2 -> Relational Operator3/2, Relational Operator5/1
  Relational Operator3/1 -> Gain6/1
  Relational Operator5/1 -> Bitwise Operator1/3
  Gain6/1 -> Bitwise Operator1/1
  Gain7/1 -> Bitwise Operator1/2

== system Lib_MCHP_BLKDEMO_Motor/Theta2PWM/Theta2PWM Optimized/Maximum Duty-Cycle ==
  In1 : Inport
  Constant1 : Constant  Value=PWMmax  OutDataTypeStr=uint16
  MinMax1 : MinMax  Function=max  OutDataTypeStr=int16  InputSameDT=on
  Sum1 : Sum  Inputs=+-  AccumDataTypeStr=uint16  OutDataTypeStr=Inherit: Same as accumulator  RndMeth=Simplest
  Sum2 : Sum  Inputs=|++  AccumDataTypeStr=uint16  OutDataTypeStr=Inherit: Same as accumulator  RndMeth=Simplest
  Out1 : Outport
  wires:
  Constant1/1 -> Sum1/1
  MinMax1/1 -> Sum1/2
  In1/1 -> Sum2/1, MinMax1/1
  Sum2/1 -> Out1/1
  Sum1/1 -> Sum2/2

== system Lib_MCHP_BLKDEMO_Motor/Theta2PWM/Theta2PWM Optimized/Minimum Duty-Cycle ==
  In1 : Inport
  Bias : Bias  Bias=-round( (2e-6/5e-5) *PWMmax )
  MinMax1 : MinMax  OutDataTypeStr=int16  InputSameDT=on
  Sum2 : Sum  Inputs=|+-  AccumDataTypeStr=uint16  OutDataTypeStr=Inherit: Same as accumulator  RndMeth=Simplest
  Out1 : Outport
  wires:
  In1/1 -> MinMax1/1, Sum2/1
  Sum2/1 -> Out1/1
  MinMax1/1 -> Bias/1
  Bias/1 -> Sum2/2

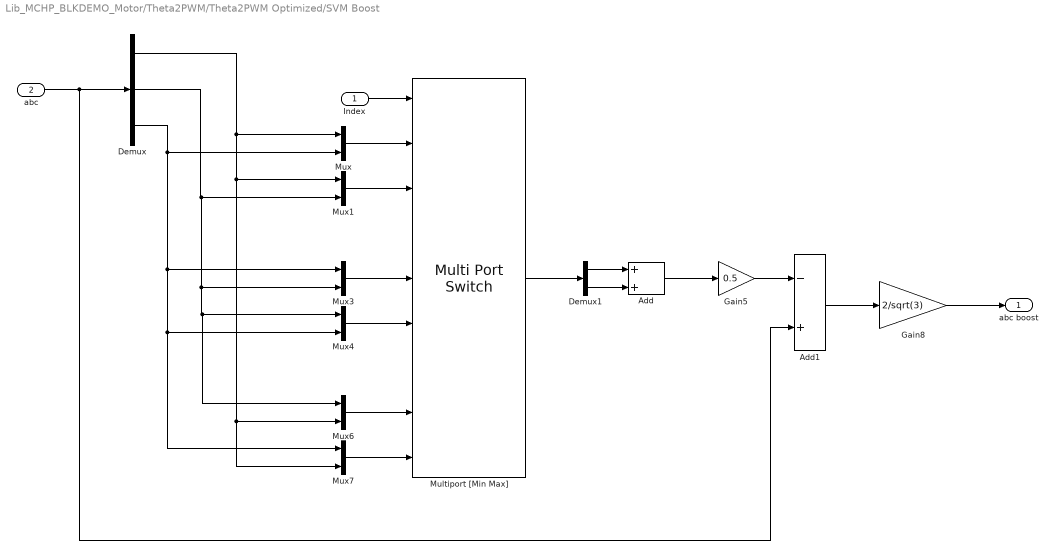
== system Lib_MCHP_BLKDEMO_Motor/Theta2PWM/Theta2PWM Optimized/SVM Boost ==
  Index : Inport
  abc : Inport  Port=2
  Add : Sum  OutDataTypeStr=Inherit: Same as accumulator  RndMeth=Simplest
  Add1 : Sum  Inputs=-+  OutDataTypeStr=Inherit: Same as accumulator  RndMeth=Simplest
  Demux : Demux  Outputs=3
  Demux1 : Demux  Outputs=2
  Gain5 : Gain  Gain=0.5  RndMeth=Simplest  OutDataTypeStr=Inherit: Same as input
  Gain8 : Gain  Gain=2/sqrt(3)  RndMeth=Simplest  OutDataTypeStr=Inherit: Same as input
  Multiport [Min Max] : MultiPortSwitch  DataPortOrder=Zero-based contiguous  Inputs=8  DiagnosticForDefault=None
  Mux{,1,3..4,6..7} (6 alike) : Mux  Inputs=2
  abc boost : Outport
  wires:
  Add/1 -> Gain5/1
  Gain5/1 -> Add1/1
  Add1/1 -> Gain8/1
  abc/1 -> Add1/2, Demux/1
  Gain8/1 -> abc boost/1
  Index/1 -> Multiport [Min Max]/1
  Mux/1 -> Multiport [Min Max]/2
  Mux1/1 -> Multiport [Min Max]/3
  Mux3/1 -> Multiport [Min Max]/5
  Mux4/1 -> Multiport [Min Max]/6
  Mux6/1 -> Multiport [Min Max]/8
  Mux7/1 -> Multiport [Min Max]/9
  Demux/1 -> Mux7/2, Mux6/2, Mux1/1, Mux/1
  Demux/3 -> Mux/2, Mux3/1, Mux4/2, Mux7/1
  Demux/2 -> Mux6/1, Mux4/1, Mux3/2, Mux1/2
  Multiport [Min Max]/1 -> Demux1/1
  Demux1/1 -> Add/1
  Demux1/2 -> Add/2

== system Lib_MCHP_BLKDEMO_Motor/Theta2PWM/Theta2PWM Optimized/Sine Simpler ==
  note: Gain is about 2us (70 MIPS)
  Theta : Inport
  Bias1 : Bias  Bias=0.25
  Look-Up Table (sin) : Lookup_n-D  NumberOfTableDimensions=1  BreakpointsSpecification=Even spacing  BreakpointsForDimension1=XData  BreakpointsForDimension1FirstPoint=0  BreakpointsForDimension1Spacing=2^-8  IndexSearchMethod=Evenly spaced points  Table="fix( 2^15 * sin(2*pi* ([0:2^-8:(1-2^-8)]+2^-9 ) )   ) * 2^-15"  InterpMethod=Flat  ExtrapMethod=Clip  RemoveProtectionInput=on  InternalRulePriority=Speed  OutDataTypeStr=fixdt(1, 16, 14)  RndMeth=Simplest  LockScale=on
  Look-Up Table (sin)1 : Lookup_n-D  NumberOfTableDimensions=1  BreakpointsSpecification=Even spacing  BreakpointsForDimension1=XData  BreakpointsForDimension1FirstPoint=0  BreakpointsForDimension1Spacing=2^-8  IndexSearchMethod=Evenly spaced points  Table="fix( 2^15 * sin(2*pi* ([0:2^-8:(1-2^-8)]+2^-9 ) )   ) * 2^-15"  InterpMethod=Flat  ExtrapMethod=Clip  RemoveProtectionInput=on  InternalRulePriority=Speed  OutDataTypeStr=fixdt(1, 16, 14)  RndMeth=Simplest  LockScale=on
  Sine1 : simulink/Lookup Tables/Sine  Formula=sin(2*pi*u) and cos(2*pi*u)  NumDataPoints=(2^5)+1  OutputWordLength=16  InternalRulePriority=Speed
  cos(2*pi*u) : Outport
  sin(2*pi*u) : Outport  Port=2
  wires:
  Look-Up Table (sin)1/1 -> cos(2*pi*u)/1
  Look-Up Table (sin)/1 -> sin(2*pi*u)/1
  Theta/1 -> Sine1/1, Look-Up Table (sin)/1, Bias1/1
  Bias1/1 -> Look-Up Table (sin)1/1

== system Lib_MCHP_BLKDEMO_Motor/Theta2PWM/Theta2PWM Optimized/inv Clark ==
  note: Transposed version is better optimized with DSP (optional)
      | No impact on no DSP version
  note: k = 2/3 : invariant Magnitude
  alpha beta : Inport
  Clarke1 : Product  Multiplication=Matrix(*)  RndMeth=Simplest  OutDataTypeStr=Inherit: Same as first input
  Constant Magnitude : Constant  Value=[1 0 ; -1/2 sqrt(3)/2 ;-1/2 -sqrt(3)/2]'  OutDataTypeStr=Inherit: Inherit via back propagation  SampleTime=-1
  Demux : Demux  Outputs=2
  Gain : Gain  Gain=sqrt(3)/2  OutDataTypeStr=Inherit: Same as input
  Gain3 : Gain  Gain=-1/2  RndMeth=Simplest  OutDataTypeStr=Inherit: Same as input
  Math Function : Math  Operator=transpose  SaturateOnIntegerOverflow=on
  Mux : Mux  Inputs=3
  Sum : Sum  RndMeth=Simplest  OutDataTypeStr=Inherit: Same as first input
  Sum1 : Sum  Inputs=+-  RndMeth=Simplest  OutDataTypeStr=Inherit: Same as first input
  abc : Outport
  wires:
  Constant Magnitude/1 -> Clarke1/2
  alpha beta/1 -> Demux/1, Math Function/1
  Math Function/1 -> Clarke1/1
  Demux/1 -> Gain3/1, Mux/1
  Demux/2 -> Gain/1
  Gain/1 -> Sum/1, Sum1/2
  Sum/1 -> Mux/2
  Sum1/1 -> Mux/3
  Mux/1 -> abc/1
  Gain3/1 -> Sum1/1, Sum/2

== system Lib_MCHP_BLKDEMO_Motor/MOTOR/DUAL SHUNT Center Aligned/MOTOR - Board Sensor/encoder scaled ==
  Rst : Inport
  Direct Lookup Table (n-D) : LookupNDDirect  NumberOfTableDimensions=1  Table=[0:199]*inv(200)  TableDataTypeStr=fixdt(0,16,16)
      settings: LockScale=on
  Q0.4 : DataTypeConversion
  QEI : MCHP_Blockset/QEI/QEI  QEI_REF=1  QEI_MODE=Quadrature Encoder  QEI_x2mode=off  QEI_PulseCountDir=Down  PIN_QEA=Dynamic Options  PIN_QEA_TXT=C6 / P54 / Pin[50]  PIN_QEB=Dynamic Options  PIN_QEB_TXT=F0 / P96 / Pin[58]  SWPAB=on  QEAPOL=off  QEBPOL=off  SampleTime=-1  INDXxCNT_Output=is not an output  POSxCNT_Output=is a 16 bits unsigned block output  RESET_Input=on  PIMOD_mode=position is cyclique between user defined boundaries  PIMOD_modeB=Never reset position  PIMOD_reset=on next INDEX event  PIN_INDEX=Dynamic Options  PIN_INDEX_TXT=B15 / P47 / Pin[3]  IMV=QEA = 1 and QEB = 0  IMV_x2=QEA = 1  PIN_HOME=Dynamic Options  PIN_HOME_TXT=B9 / P41 / Pin[49]  QEIxLEC_GEC=[0 199]  QEIxIC=0  PCIIRQ=off  IDXPOL=off  HOMPOL=on  VELxCNT_Output=is not an output  INTxHLD_Output=is not an output  MaxPeriod=0.1  FILTREN=on  QFDIV_popup=Dynamic Options  QFDIV_popup_TXT=364.58 kHz  FILTER_CutOffFreq=100e3  PIN_CCMP=Dynamic Options  PIN_CCMP_TXT=A4 / P20 / Pin[33]  MCHP_PORT={QEI1 A}{QEA1}5:0:P54;{QEI1 B}{QEB1}5:0:P96;  MCHP_MASTERLINK=AN1078_33EP256MC506_ClosedLoop/Microchip Master  QEI_IntPri=5
  Rate Transition4 : RateTransition  X0=1
  theta_enc_fract : Outport
  wires:
  QEI/1 -> Direct Lookup Table (n-D)/1
  Direct Lookup Table (n-D)/1 -> theta_enc_fract/1
  Rst/1 -> Q0.4/1
  Q0.4/1 -> Rate Transition4/1
  Rate Transition4/1 -> QEI/1

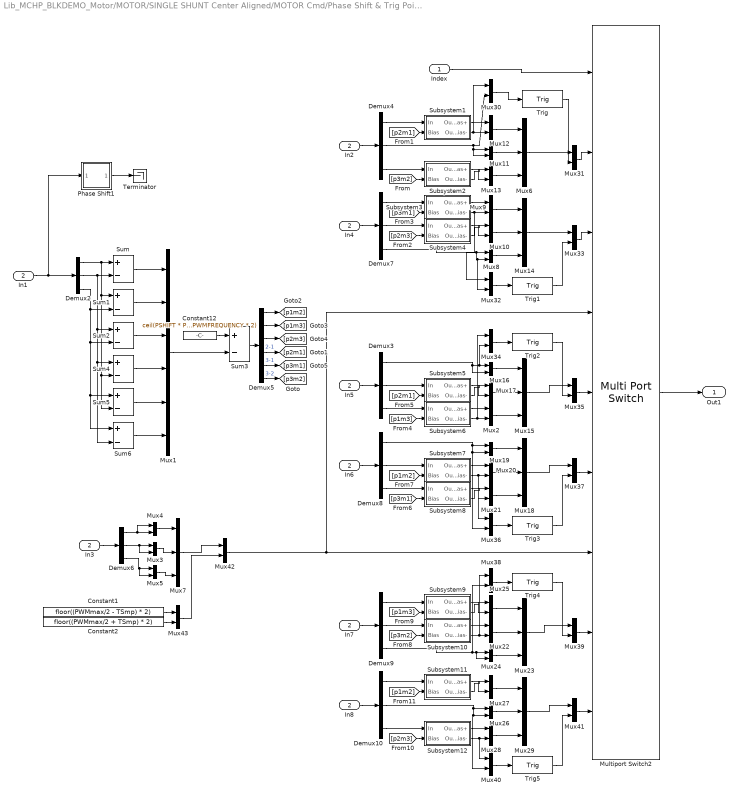
== system Lib_MCHP_BLKDEMO_Motor/MOTOR/SINGLE SHUNT Center Aligned/MOTOR Cmd/Phase Shift & Trig Point ==
  Index : Inport
  In1 : Inport  Port=2
  Constant1 : Constant  Value=floor((PWMmax/2 - TSmp) * 2)  OutDataTypeStr=uint16
  Constant12 : Constant  Value=ceil(PSHIFT * PWMmax * PWMFREQUENCY * 2)  OutDataTypeStr=uint16
  Constant2 : Constant  Value=floor((PWMmax/2 + TSmp) * 2)  OutDataTypeStr=uint16
  Demux{2..4,6..10} (8 alike) : Demux  Outputs=3
  Demux5 : Demux  Outputs=6
  In{2..8} (7 alike) : InportShadow  Port=2
  Multiport Switch2 : MultiPortSwitch  DataPortOrder=Zero-based contiguous  Inputs=8  DiagnosticForDefault=None
  Mux1 : Mux  Inputs=6
  Mux{2..5,8..13,16..17,19..22,24..28,30..43} (35 alike) : Mux  Inputs=2
  Mux{6..7,14..15,18,23,29} (7 alike) : Mux  Inputs=3
  Phase Shift1 : Subsystem
  Subsystem1 : Subsystem
  Subsystem10 : Subsystem
  Subsystem11 : Subsystem
  Subsystem12 : Subsystem
  Subsystem2 : Subsystem
  Subsystem3 : Subsystem
  Subsystem4 : Subsystem
  Subsystem5 : Subsystem
  Subsystem6 : Subsystem
  Subsystem7 : Subsystem
  Subsystem8 : Subsystem
  Subsystem9 : Subsystem
  Sum{,1..2,4..6} (6 alike) : Sum  Inputs=+-
  Sum3 : Sum  Inputs=+-  OutDataTypeStr=Inherit: Same as accumulator  SaturateOnIntegerOverflow=on
  Terminator : Terminator
  Trig{,1..5} (6 alike) : Lib_MCHP_BLKDEMO_Motor/Internal/Trig
  Out1 : Outport
  wires:
  In1/1 -> Phase Shift1/1(In1), Demux2/1
  Demux2/1 -> Sum5/2, Sum4/2, Sum1/1, Sum/1
  Demux2/2 -> Sum6/2, Sum4/1, Sum2/1, Sum/2
  Demux2/3 -> Sum6/1, Sum5/1, Sum2/2, Sum1/2
  Sum/1 -> Mux1/1
  Sum1/1 -> Mux1/2
  Sum2/1 -> Mux1/3
  Multiport Switch2/1 -> Out1/1
  Sum4/1 -> Mux1/4
  Sum5/1 -> Mux1/5
  Sum6/1 -> Mux1/6
  Mux1/1 -> Sum3/2
  Constant12/1 -> Sum3/1
  In2/1 -> Demux4/1
  Sum3/1 -> Demux5/1
  Demux4/3 -> Subsystem2/1(In)
  Demux4/1 -> Subsystem1/1(In)
  Demux4/2 -> Mux11/2, Mux11/1, Mux30/2
  Mux12/1 -> Mux6/1
  Mux11/1 -> Mux6/2
  Mux13/1 -> Mux6/3
  Demux6/2 -> Mux3/2, Mux3/1
  In3/1 -> Demux6/1
  Demux6/1 -> Mux4/1, Mux4/2
  Demux6/3 -> Mux5/2, Mux5/1
  Mux4/1 -> Mux7/1
  Mux3/1 -> Mux7/2
  Mux5/1 -> Mux7/3
  Mux42/1 -> Multiport Switch2/4, Multiport Switch2/7
  Demux5/6 -> [p3m2]  "3-2"
  [p3m2] -> Subsystem2/2(Bias)
  Demux5/4 -> [p2m1]  "2-1"
  [p2m1] -> Subsystem1/2(Bias)
  Demux5/1 -> [p1m2]
  Demux5/5 -> [p3m1]  "3-1"
  Demux5/3 -> [p2m3]
  Demux5/2 -> [p1m3]
  In4/1 -> Demux7/1
  Demux7/2 -> Subsystem4/1(In)
  Demux7/1 -> Subsystem3/1(In)
  Mux9/1 -> Mux14/1
  [p2m3] -> Subsystem4/2(Bias)
  [p3m1] -> Subsystem3/2(Bias)
  Mux8/1 -> Mux14/3
  Mux10/1 -> Mux14/2
  Demux7/3 -> Mux32/2, Mux8/2, Mux8/1
  In5/1 -> Demux3/1
  [p1m3] -> Subsystem6/2(Bias)
  [p2m1] -> Subsystem5/2(Bias)
  Demux3/3 -> Subsystem6/1(In)
  Demux3/2 -> Subsystem5/1(In)
  Demux3/1 -> Mux16/2, Mux34/2, Mux16/1
  Mux16/1 -> Mux15/1
  Mux17/1 -> Mux15/2
  Mux2/1 -> Mux15/3
  In6/1 -> Demux8/1
  [p3m1] -> Subsystem8/2(Bias)
  [p1m2] -> Subsystem7/2(Bias)
  Demux8/3 -> Subsystem8/1(In)
  Demux8/2 -> Subsystem7/1(In)
  Demux8/1 -> Mux19/1, Mux36/2, Mux19/2
  Mux19/1 -> Mux18/1
  Mux20/1 -> Mux18/2
  Mux21/1 -> Mux18/3
  In7/1 -> Demux9/1
  Demux9/2 -> Subsystem10/1(In)
  Demux9/1 -> Subsystem9/1(In)
  Mux25/1 -> Mux23/1
  [p3m2] -> Subsystem10/2(Bias)
  [p1m3] -> Subsystem9/2(Bias)
  Mux24/1 -> Mux23/3
  Mux22/1 -> Mux23/2
  Demux9/3 -> Mux24/1, Mux24/2, Mux38/2
  In8/1 -> Demux10/1
  Demux10/3 -> Subsystem12/1(In)
  Demux10/1 -> Subsystem11/1(In)
  Demux10/2 -> Mux40/2, Mux26/2, Mux26/1
  Mux27/1 -> Mux29/1
  Mux26/1 -> Mux29/2
  Mux28/1 -> Mux29/3
  [p2m3] -> Subsystem12/2(Bias)
  [p1m2] -> Subsystem11/2(Bias)
  Subsystem12/1(Out bias+) -> Mux28/1
  Subsystem12/2(Out bias-) -> Mux40/1, Mux28/2
  Subsystem11/1(Out bias+) -> Mux27/2
  Subsystem11/2(Out bias-) -> Mux27/1
  Subsystem1/1(Out bias+) -> Mux12/1
  Subsystem1/2(Out bias-) -> Mux30/1, Mux12/2
  Subsystem2/1(Out bias+) -> Mux13/2
  Subsystem2/2(Out bias-) -> Mux13/1
  Subsystem3/1(Out bias+) -> Mux9/1
  Subsystem3/2(Out bias-) -> Mux32/1, Mux9/2
  Subsystem4/1(Out bias+) -> Mux10/2
  Subsystem4/2(Out bias-) -> Mux10/1
  Subsystem6/1(Out bias+) -> Mux2/1
  Subsystem6/2(Out bias-) -> Mux34/1, Mux2/2
  Subsystem5/1(Out bias+) -> Mux17/2
  Subsystem5/2(Out bias-) -> Mux17/1
  Subsystem7/1(Out bias+) -> Mux20/1
  Subsystem7/2(Out bias-) -> Mux36/1, Mux20/2
  Subsystem8/1(Out bias+) -> Mux21/2
  Subsystem8/2(Out bias-) -> Mux21/1
  Subsystem10/1(Out bias+) -> Mux22/1
  Subsystem10/2(Out bias-) -> Mux38/1, Mux22/2
  Subsystem9/1(Out bias+) -> Mux25/2
  Subsystem9/2(Out bias-) -> Mux25/1
  Mux30/1 -> Trig/1
  Mux31/1 -> Multiport Switch2/2
  Mux6/1 -> Mux31/1
  Trig/1 -> Mux31/2
  Mux32/1 -> Trig1/1
  Mux14/1 -> Mux33/1
  Mux33/1 -> Multiport Switch2/3
  Trig1/1 -> Mux33/2
  Mux34/1 -> Trig2/1
  Mux35/1 -> Multiport Switch2/5
  Mux15/1 -> Mux35/1
  Trig2/1 -> Mux35/2
  Mux36/1 -> Trig3/1
  Mux18/1 -> Mux37/1
  Mux37/1 -> Multiport Switch2/6
  Trig3/1 -> Mux37/2
  Mux38/1 -> Trig4/1
  Trig4/1 -> Mux39/2
  Mux40/1 -> Trig5/1
  Trig5/1 -> Mux41/2
  Mux39/1 -> Multiport Switch2/8
  Mux41/1 -> Multiport Switch2/9
  Mux29/1 -> Mux41/1
  Mux23/1 -> Mux39/1
  Mux7/1 -> Mux42/1
  Constant1/1 -> Mux43/1
  Constant2/1 -> Mux43/2
  Mux43/1 -> Mux42/2
  Index/1 -> Multiport Switch2/1
  Phase Shift1/1(Out1) -> Terminator/1

== system Lib_MCHP_BLKDEMO_Motor/MOTOR/SINGLE SHUNT Center Aligned/MOTOR - Board Sensor/Reconstruct Ia Ib ==
  Index : Inport
  I : Inport  Port=2
  Demux3 : Demux  Outputs=2
  Gain1 : Gain  Gain=-1  OutDataTypeStr=Inherit: Same as input
  Multiport Switch1 : MultiPortSwitch  DataPortOrder=Zero-based contiguous  Inputs=8  DiagnosticForDefault=None
  Multiport Switch2 : MultiPortSwitch  DataPortOrder=Zero-based contiguous  Inputs=8  DiagnosticForDefault=None
  Mux : Mux  Inputs=2
  Sum1 : Sum  Inputs=+-
  Ia Ib : Outport
  wires:
  I/1 -> Demux3/1
  Index/1 -> Multiport Switch1/1, Multiport Switch2/1
  Demux3/1 -> Multiport Switch2/6, Multiport Switch2/8, Multiport Switch1/3, Multiport Switch1/2, Sum1/2
  Demux3/2 -> Gain1/1, Sum1/1
  Mux/1 -> Ia Ib/1
  Multiport Switch2/1 -> Mux/2
  Multiport Switch1/1 -> Mux/1
  Gain1/1 -> Multiport Switch2/5, Multiport Switch2/3, Multiport Switch1/9, Multiport Switch1/8
  Sum1/1 -> Multiport Switch1/5, Multiport Switch1/6, Multiport Switch2/2, Multiport Switch2/9

== system Lib_MCHP_BLKDEMO_Motor/MOTOR/SINGLE SHUNT Center Aligned/MOTOR - Board Sensor/encoder scaled ==
  Rst : Inport
  Direct Lookup Table (n-D) : LookupNDDirect  NumberOfTableDimensions=1  Table=[0:199]*inv(200)  TableDataTypeStr=fixdt(0,16,16)
      settings: LockScale=on
  Q0.4 : DataTypeConversion
  QEI : MCHP_Blockset/QEI/QEI  QEI_REF=1  QEI_MODE=Quadrature Encoder  QEI_x2mode=off  QEI_PulseCountDir=Down  PIN_QEA=Dynamic Options  PIN_QEA_TXT=C6 / P54 / Pin[50]  PIN_QEB=Dynamic Options  PIN_QEB_TXT=F0 / P96 / Pin[58]  SWPAB=on  QEAPOL=off  QEBPOL=off  SampleTime=-1  INDXxCNT_Output=is not an output  POSxCNT_Output=is a 16 bits unsigned block output  RESET_Input=on  PIMOD_mode=position is cyclique between user defined boundaries  PIMOD_modeB=Never reset position  PIMOD_reset=on next INDEX event  PIN_INDEX=Dynamic Options  PIN_INDEX_TXT=B15 / P47 / Pin[3]  IMV=QEA = 1 and QEB = 0  IMV_x2=QEA = 1  PIN_HOME=Dynamic Options  PIN_HOME_TXT=B9 / P41 / Pin[49]  QEIxLEC_GEC=[0 199]  QEIxIC=0  PCIIRQ=off  IDXPOL=off  HOMPOL=on  VELxCNT_Output=is not an output  INTxHLD_Output=is not an output  MaxPeriod=0.1  FILTREN=on  QFDIV_popup=Dynamic Options  QFDIV_popup_TXT=364.58 kHz  FILTER_CutOffFreq=100e3  PIN_CCMP=Dynamic Options  PIN_CCMP_TXT=A4 / P20 / Pin[33]  MCHP_PORT={QEI1 A}{QEA1}5:0:P54;{QEI1 B}{QEB1}5:0:P96;  MCHP_MASTERLINK=Test_PWMHS_33EP256MC506/Microchip Master  QEI_IntPri=5
  Rate Transition4 : RateTransition  X0=1
  theta_enc_fract : Outport
  wires:
  Rate Transition4/1 -> QEI/1
  Q0.4/1 -> Rate Transition4/1
  Rst/1 -> Q0.4/1
  Direct Lookup Table (n-D)/1 -> theta_enc_fract/1
  QEI/1 -> Direct Lookup Table (n-D)/1

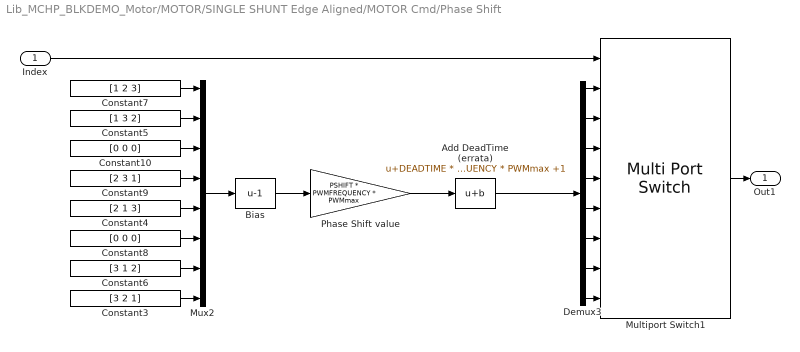
== system Lib_MCHP_BLKDEMO_Motor/MOTOR/SINGLE SHUNT Edge Aligned/MOTOR Cmd/Phase Shift ==
  Index : Inport
  Add DeadTime (errata) : Bias  Bias=DEADTIME * PWMFREQUENCY * PWMmax +1
  Bias : Bias  Bias=-1
  Constant10 : Constant  Value=[0 0 0]  OutDataTypeStr=int16
  Constant3 : Constant  Value=[3 2 1]  OutDataTypeStr=int16
  Constant4 : Constant  Value=[2 1 3]  OutDataTypeStr=int16
  Constant5 : Constant  Value=[1 3 2]  OutDataTypeStr=int16
  Constant6 : Constant  Value=[3 1 2]  OutDataTypeStr=int16
  Constant7 : Constant  Value=[1 2 3]  OutDataTypeStr=int16
  Constant8 : Constant  Value=[0 0 0]  OutDataTypeStr=int16
  Constant9 : Constant  Value=[2 3 1]  OutDataTypeStr=int16
  Demux3 : Demux  Outputs=8
  Multiport Switch1 : MultiPortSwitch  DataPortOrder=Zero-based contiguous  Inputs=8  DiagnosticForDefault=None
  Mux2 : Mux  Inputs=8
  Phase Shift value : Gain  Gain=PSHIFT * PWMFREQUENCY * PWMmax  OutDataTypeStr=uint16  SaturateOnIntegerOverflow=on
  Out1 : Outport
  wires:
  Index/1 -> Multiport Switch1/1
  Demux3/2 -> Multiport Switch1/3
  Demux3/8 -> Multiport Switch1/9
  Demux3/5 -> Multiport Switch1/6
  Demux3/3 -> Multiport Switch1/4
  Demux3/7 -> Multiport Switch1/8
  Demux3/4 -> Multiport Switch1/5
  Mux2/1 -> Bias/1
  Demux3/1 -> Multiport Switch1/2
  Phase Shift value/1 -> Add DeadTime (errata)/1
  Demux3/6 -> Multiport Switch1/7
  Multiport Switch1/1 -> Out1/1
  Constant7/1 -> Mux2/1
  Constant5/1 -> Mux2/2
  Constant10/1 -> Mux2/3
  Constant9/1 -> Mux2/4
  Constant4/1 -> Mux2/5
  Constant8/1 -> Mux2/6
  Constant6/1 -> Mux2/7
  Constant3/1 -> Mux2/8
  Bias/1 -> Phase Shift value/1
  Add DeadTime (errata)/1 -> Demux3/1

== system Lib_MCHP_BLKDEMO_Motor/MOTOR/SINGLE SHUNT Edge Aligned/MOTOR - Board Sensor/Reconstruct Ia Ib ==
  Index : Inport
  I : Inport  Port=2
  Demux3 : Demux  Outputs=2
  Gain1 : Gain  Gain=-1  OutDataTypeStr=Inherit: Same as input
  Multiport Switch1 : MultiPortSwitch  DataPortOrder=Zero-based contiguous  Inputs=8  DiagnosticForDefault=None
  Multiport Switch2 : MultiPortSwitch  DataPortOrder=Zero-based contiguous  Inputs=8  DiagnosticForDefault=None
  Mux : Mux  Inputs=2
  Sum1 : Sum  Inputs=+-
  Ia Ib : Outport
  wires:
  I/1 -> Demux3/1
  Index/1 -> Multiport Switch1/1, Multiport Switch2/1
  Demux3/1 -> Multiport Switch2/6, Multiport Switch2/8, Multiport Switch1/3, Multiport Switch1/2, Sum1/2
  Demux3/2 -> Gain1/1, Sum1/1
  Mux/1 -> Ia Ib/1
  Multiport Switch2/1 -> Mux/2
  Multiport Switch1/1 -> Mux/1
  Gain1/1 -> Multiport Switch2/5, Multiport Switch2/3, Multiport Switch1/9, Multiport Switch1/8
  Sum1/1 -> Multiport Switch1/5, Multiport Switch1/6, Multiport Switch2/2, Multiport Switch2/9
